simulink model "sensorExpoler_Encoder_Bourns"  (R2026a)
settings: Solver=FixedStepDiscrete  StopTime=32  FixedStep=0.0001
undefined symbols (not defined in the file): Blocking, Non
libraries: amg_usbconverter_n_connect_lib x2
settings Model: Creator=pboon  LastModifiedBy=matthurindo

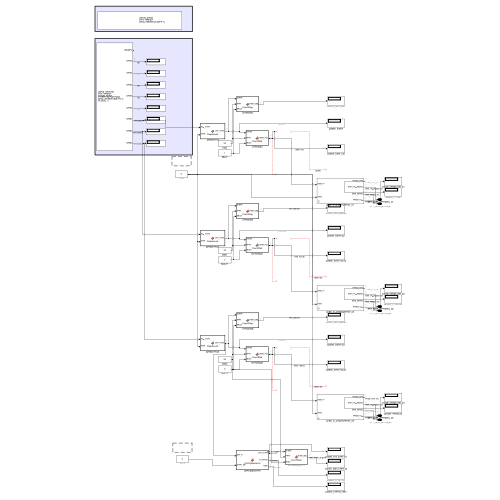
[thumbnail: Simulink's stored preview of the top-level diagram]
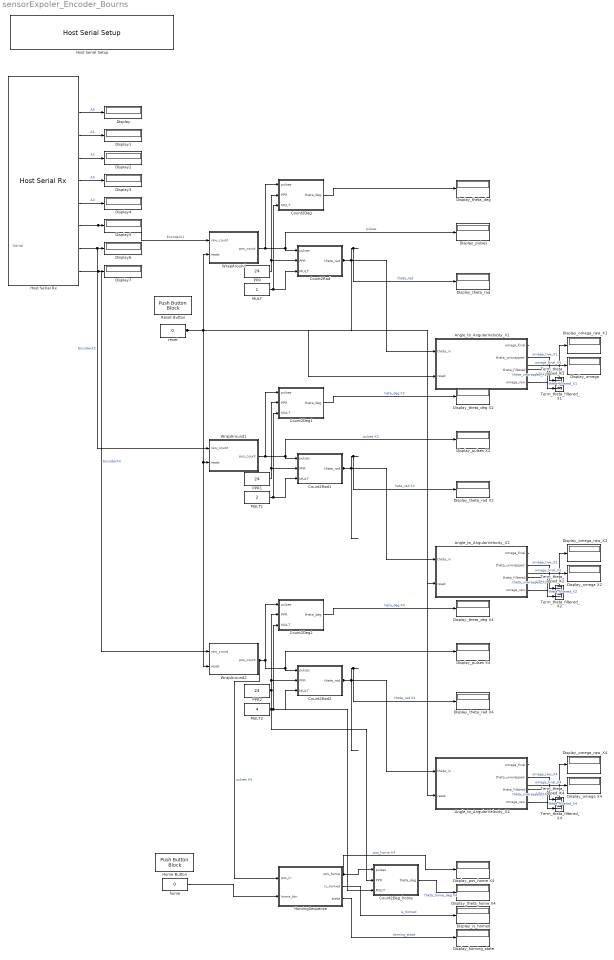
== system sensorExpoler_Encoder_Bourns ==
  note: Serial
  Angle_to_AngularVelocity_X1 : Subsystem  mask{Ts=0.001, fc_theta=0.5, fc_omega=5, Enable_velocity_filter=1, Enable_unwrap=0, Wrap_period=2*pi}
      mask prompts: Ts "Effective sensor sample time [s]"; fc_theta "Angle low-pass cutoff [Hz] (0 < fc < 1/(2*Ts))"; fc_omega "Velocity low-pass cutoff [Hz]"; Enable_velocity_filter "1 = light velocity LPF on, 0 = bypass"; Enable_unwrap "1 = unwrap a wrapped angle, 0 = angle already accumulated"; Wrap_period "Wrap period [rad] (2*pi) or [deg] (360)"
      mask help:
      | Filtered angle -> angular velocity (X1).
      | theta -> [unwrap] -> [1st-order angle LPF @ fc_theta] -> [(theta[k]-theta[k-1])/Ts] -> [light velocity LPF @ fc_omega] -> omega.
      | State initialised from the first valid sample; output 0 on first sample/reset.
  Angle_to_AngularVelocity_X2 : Subsystem  mask{Ts=0.001, fc_theta=1, fc_omega=5, Enable_velocity_filter=1, Enable_unwrap=0, Wrap_period=2*pi}
      mask prompts: Ts "Effective sensor sample time [s]"; fc_theta "Angle low-pass cutoff [Hz] (0 < fc < 1/(2*Ts))"; fc_omega "Velocity low-pass cutoff [Hz]"; Enable_velocity_filter "1 = light velocity LPF on, 0 = bypass"; Enable_unwrap "1 = unwrap a wrapped angle, 0 = angle already accumulated"; Wrap_period "Wrap period [rad] (2*pi) or [deg] (360)"
      mask help:
      | Filtered angle -> angular velocity (X2).
      | theta -> [unwrap] -> [1st-order angle LPF @ fc_theta] -> [(theta[k]-theta[k-1])/Ts] -> [light velocity LPF @ fc_omega] -> omega.
      | State initialised from the first valid sample; output 0 on first sample/reset.
  Angle_to_AngularVelocity_X4 : Subsystem  mask{Ts=0.001, fc_theta=2, fc_omega=5, Enable_velocity_filter=1, Enable_unwrap=0, Wrap_period=2*pi}
      mask prompts: Ts "Effective sensor sample time [s]"; fc_theta "Angle low-pass cutoff [Hz] (0 < fc < 1/(2*Ts))"; fc_omega "Velocity low-pass cutoff [Hz]"; Enable_velocity_filter "1 = light velocity LPF on, 0 = bypass"; Enable_unwrap "1 = unwrap a wrapped angle, 0 = angle already accumulated"; Wrap_period "Wrap period [rad] (2*pi) or [deg] (360)"
      mask help:
      | Filtered angle -> angular velocity (X4).
      | theta -> [unwrap] -> [1st-order angle LPF @ fc_theta] -> [(theta[k]-theta[k-1])/Ts] -> [light velocity LPF @ fc_omega] -> omega.
      | State initialised from the first valid sample; output 0 on first sample/reset.
  Count2Deg : MATLAB Function  TreatAsAtomicUnit=on
  Count2Deg1 : MATLAB Function  TreatAsAtomicUnit=on
  Count2Deg2 : MATLAB Function  TreatAsAtomicUnit=on
  Count2Deg_home : MATLAB Function  TreatAsAtomicUnit=on
  Count2Rad : MATLAB Function  TreatAsAtomicUnit=on
  Count2Rad1 : MATLAB Function  TreatAsAtomicUnit=on
  Count2Rad2 : MATLAB Function  TreatAsAtomicUnit=on
  Display{,1..7} (8 alike) : Display
  Display_homing_state : Display
  Display_is_homed : Display
  Display_omega : Display
  Display_omega X2 : Display
  Display_omega X4 : Display
  Display_omega_raw_X1 : Display
  Display_omega_raw_X2 : Display
  Display_omega_raw_X4 : Display
  Display_pos_home X4 : Display
  Display_pulses : Display
  Display_pulses X2 : Display
  Display_pulses X4 : Display
  Display_theta_deg : Display
  Display_theta_deg X2 : Display
  Display_theta_deg X4 : Display
  Display_theta_home X4 : Display
  Display_theta_rad : Display
  Display_theta_rad X2 : Display
  Display_theta_rad X4 : Display
  Home Button : PushButtonBlock  ButtonText=Home  IconOnColor=[0.0, 0.39215686274509803, 0.0]  IconOffColor=[0.0, 1.0, 0.0]  OffValue=0.000000
  HomingSequence : MATLAB Function  TreatAsAtomicUnit=on
  Host Serial Rx : amg_usbconverter_n_connect_lib/Host Serial Rx  conf=rx  port=<auto>  baudrate=2000000  databits=8  parity=None  stopbit=1  flowcontrol=None  transfer=Non-Blocking  timeout=5  packetmode=Binary  enableinitialvalues=off  initialvalues=[]  binheader='25'  binterminator='4E 4E'  porttype_double=0  porttype_single=0  porttype_int8=0  porttype_uint8=0  porttype_int16=0  porttype_uint16=5  porttype_int32=0  porttype_uint32=3  asciiformat='%d,%f'  rx_asciiterminator="CRLF (0x0D 0x0A - \"\\r\\n\")"  tx_asciiterminator="CRLF (0x0D 0x0A - \"\\r\\n\")"  sampletime=0.001  enablecustomportlabel=off  cinputportlabel=0  coutputportlabel=A  portpinstr=0  blockid=HostSerialRx  inputporttype=[]  inputportwidth=[]  inputportlabel={}  outputporttype=[3 5 5 5 5 5 7 7 7]  outputportwidth=[1 1 1 1 1 1 1 1 1]  outputportlabel={'READY','uint16','uint16','uint16','uint16','uint16','uint32','uint32','uint32'}  compat=0  optionstring=[]  autoport='<empty>'
  Host Serial Setup : amg_usbconverter_n_connect_lib/Host Serial Setup  conf=setup  port=<auto>  baudrate=2000000  databits=8  parity=None  stopbit=1  flowcontrol=None  transfer=Blocking  timeout=2  packetmode=Binary  initialvalues=[]  binheader='7E 7E'  binterminator='03 03'  porttype_double=0  porttype_single=1  porttype_int8=0  porttype_uint8=0  porttype_int16=0  porttype_uint16=0  porttype_int32=0  porttype_uint32=2  asciiformat='%d %u %x'  rx_asciiterminator="CRLF (0x0D 0x0A - \"\\r\\n\")"  tx_asciiterminator="CRLF (0x0D 0x0A - \"\\r\\n\")"  sampletime=-1  enablecustomportlabel=off  cinputportlabel=0  coutputportlabel=A  portpinstr=0  blockid=HostSerialSetup  inputporttype=[]  inputportwidth=[]  inputportlabel={}  outputporttype=[]  outputportwidth=[]  outputportlabel={}  compat=0  optionstring=[]  autoport='<empty>'
  MULT : Constant
  MULT1 : Constant  Value=2
  MULT2 : Constant  Value=4
  PPR : Constant  Value=24
  PPR1 : Constant  Value=24
  PPR2 : Constant  Value=24
  Reset Button : PushButtonBlock  IconOnColor=[0.0, 0.39215686274509803, 0.0]  IconOffColor=[0.0, 1.0, 0.0]  OffValue=0.000000
  Term_theta_filtered_X1 : Terminator
  Term_theta_filtered_X2 : Terminator
  Term_theta_filtered_X4 : Terminator
  Term_theta_unwrapped_X1 : Terminator
  Term_theta_unwrapped_X2 : Terminator
  Term_theta_unwrapped_X4 : Terminator
  WrapAround : MATLAB Function  TreatAsAtomicUnit=on
  WrapAround1 : MATLAB Function  TreatAsAtomicUnit=on
  WrapAround2 : MATLAB Function  TreatAsAtomicUnit=on
  home : Constant  Value=0
  reset : Constant  Value=0
  wires:
  Host Serial Rx/2 -> Display/1  "A0"
  Host Serial Rx/3 -> Display1/1  "A1"
  Host Serial Rx/4 -> Display2/1  "A2"
  Host Serial Rx/5 -> Display3/1  "A3"
  Host Serial Rx/6 -> Display4/1  "A4"
  Host Serial Rx/7 -> WrapAround/1(raw_count), Display5/1  "EncoderX1"
  Host Serial Rx/8 -> WrapAround1/1(raw_count), Display6/1  "EncoderX2"
  Host Serial Rx/9 -> WrapAround2/1(raw_count), Display7/1  "EncoderX4"
  reset/1 -> WrapAround/2(reset), WrapAround1/2(reset), WrapAround2/2(reset), Angle_to_AngularVelocity_X1/2(reset), Angle_to_AngularVelocity_X2/2(reset), Angle_to_AngularVelocity_X4/2(reset)
  PPR/1 -> Count2Rad/2(PPR), Count2Deg/2(PPR)
  MULT/1 -> Count2Rad/3(MULT), Count2Deg/3(MULT)
  WrapAround/1(pos_count) -> Count2Rad/1(pulses), Display_pulses/1, Count2Deg/1(pulses)  "pulses"
  Count2Rad/1(theta_rad) -> Display_theta_rad/1, Angle_to_AngularVelocity_X1/1(theta_in)  "theta_rad"
  Count2Deg/1(theta_deg) -> Display_theta_deg/1
  ? -> ?  "dtheta"
  ? -> ?  "dtheta X2"
  WrapAround1/1(pos_count) -> Count2Rad1/1(pulses), Display_pulses X2/1, Count2Deg1/1(pulses)  "pulses X2"
  MULT1/1 -> Count2Rad1/3(MULT), Count2Deg1/3(MULT)
  Count2Rad1/1(theta_rad) -> Display_theta_rad X2/1, Angle_to_AngularVelocity_X2/1(theta_in)  "heta_rad X2"
  Count2Deg1/1(theta_deg) -> Display_theta_deg X2/1  "heta_deg X2"
  PPR1/1 -> Count2Rad1/2(PPR), Count2Deg1/2(PPR)
  ? -> ?  "dtheta X4"
  WrapAround2/1(pos_count) -> Count2Rad2/1(pulses), Display_pulses X4/1, Count2Deg2/1(pulses), HomingSequence/1(pos_in)  "pulses X4"
  MULT2/1 -> Count2Rad2/3(MULT), Count2Deg2/3(MULT), Count2Deg_home/3(MULT)
  Count2Rad2/1(theta_rad) -> Display_theta_rad X4/1, Angle_to_AngularVelocity_X4/1(theta_in)  "theta_rad X4"
  Count2Deg2/1(theta_deg) -> Display_theta_deg X4/1  "heta_deg X4"
  PPR2/1 -> Count2Rad2/2(PPR), Count2Deg2/2(PPR), Count2Deg_home/2(PPR)
  Angle_to_AngularVelocity_X1/1(omega_final) -> Display_omega/1  "omega_final_X1"
  Angle_to_AngularVelocity_X1/4(omega_raw) -> Display_omega_raw_X1/1  "omega_raw_X1"
  Angle_to_AngularVelocity_X1/2(theta_unwrapped) -> Term_theta_unwrapped_X1/1  "theta_unwrapped_X1"
  Angle_to_AngularVelocity_X1/3(theta_filtered) -> Term_theta_filtered_X1/1  "theta_filtered_X1"
  Angle_to_AngularVelocity_X2/1(omega_final) -> Display_omega X2/1  "omega_final_X2"
  Angle_to_AngularVelocity_X2/4(omega_raw) -> Display_omega_raw_X2/1  "omega_raw_X2"
  Angle_to_AngularVelocity_X2/2(theta_unwrapped) -> Term_theta_unwrapped_X2/1  "theta_unwrapped_X2"
  Angle_to_AngularVelocity_X2/3(theta_filtered) -> Term_theta_filtered_X2/1  "theta_filtered_X2"
  Angle_to_AngularVelocity_X4/1(omega_final) -> Display_omega X4/1  "omega_final_X4"
  Angle_to_AngularVelocity_X4/4(omega_raw) -> Display_omega_raw_X4/1  "omega_raw_X4"
  Angle_to_AngularVelocity_X4/2(theta_unwrapped) -> Term_theta_unwrapped_X4/1  "theta_unwrapped_X4"
  Angle_to_AngularVelocity_X4/3(theta_filtered) -> Term_theta_filtered_X4/1  "theta_filtered_X4"
  home/1 -> HomingSequence/2(home_btn)
  HomingSequence/1(pos_home) -> Count2Deg_home/1(pulses), Display_pos_home X4/1  "pos_home X4"
  Count2Deg_home/1(theta_deg) -> Display_theta_home X4/1  "theta_home_deg X4"
  HomingSequence/2(is_homed) -> Display_is_homed/1  "is_homed"
  HomingSequence/3(state) -> Display_homing_state/1  "homing_state"

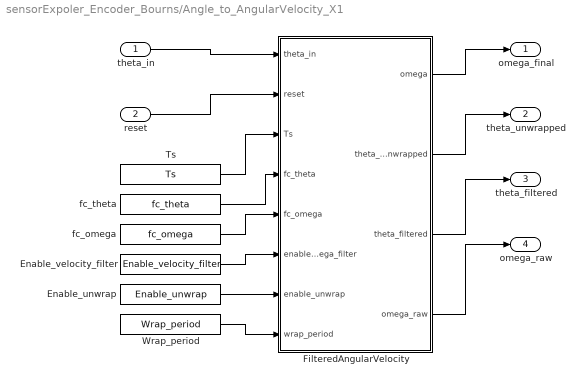
== system sensorExpoler_Encoder_Bourns/Angle_to_AngularVelocity_X1 ==
  theta_in : Inport
  reset : Inport  Port=2
  Enable_unwrap : Constant  Value=Enable_unwrap
  Enable_velocity_filter : Constant  Value=Enable_velocity_filter
  FilteredAngularVelocity : MATLAB Function  TreatAsAtomicUnit=on
  Ts : Constant  Value=Ts
  Wrap_period : Constant  Value=Wrap_period
  fc_omega : Constant  Value=fc_omega
  fc_theta : Constant  Value=fc_theta
  omega_final : Outport
  theta_unwrapped : Outport  Port=2
  theta_filtered : Outport  Port=3
  omega_raw : Outport  Port=4
  wires:
  theta_in/1 -> FilteredAngularVelocity/1(theta_in)
  reset/1 -> FilteredAngularVelocity/2(reset)
  Ts/1 -> FilteredAngularVelocity/3(Ts)
  fc_theta/1 -> FilteredAngularVelocity/4(fc_theta)
  fc_omega/1 -> FilteredAngularVelocity/5(fc_omega)
  Enable_velocity_filter/1 -> FilteredAngularVelocity/6(enable_omega_filter)
  Enable_unwrap/1 -> FilteredAngularVelocity/7(enable_unwrap)
  Wrap_period/1 -> FilteredAngularVelocity/8(wrap_period)
  FilteredAngularVelocity/1(omega) -> omega_final/1
  FilteredAngularVelocity/2(theta_unwrapped) -> theta_unwrapped/1
  FilteredAngularVelocity/3(theta_filtered) -> theta_filtered/1
  FilteredAngularVelocity/4(omega_raw) -> omega_raw/1

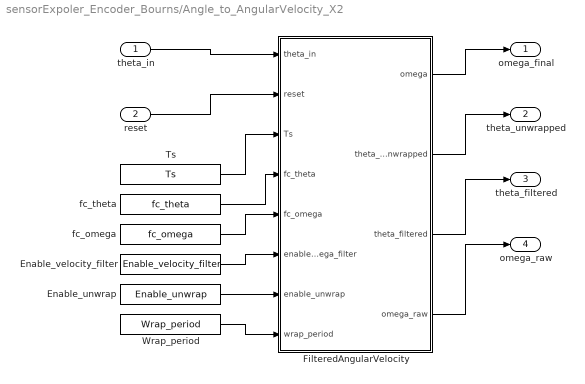
== system sensorExpoler_Encoder_Bourns/Angle_to_AngularVelocity_X2 ==
  theta_in : Inport
  reset : Inport  Port=2
  Enable_unwrap : Constant  Value=Enable_unwrap
  Enable_velocity_filter : Constant  Value=Enable_velocity_filter
  FilteredAngularVelocity : MATLAB Function  TreatAsAtomicUnit=on
  Ts : Constant  Value=Ts
  Wrap_period : Constant  Value=Wrap_period
  fc_omega : Constant  Value=fc_omega
  fc_theta : Constant  Value=fc_theta
  omega_final : Outport
  theta_unwrapped : Outport  Port=2
  theta_filtered : Outport  Port=3
  omega_raw : Outport  Port=4
  wires:
  theta_in/1 -> FilteredAngularVelocity/1(theta_in)
  reset/1 -> FilteredAngularVelocity/2(reset)
  Ts/1 -> FilteredAngularVelocity/3(Ts)
  fc_theta/1 -> FilteredAngularVelocity/4(fc_theta)
  fc_omega/1 -> FilteredAngularVelocity/5(fc_omega)
  Enable_velocity_filter/1 -> FilteredAngularVelocity/6(enable_omega_filter)
  Enable_unwrap/1 -> FilteredAngularVelocity/7(enable_unwrap)
  Wrap_period/1 -> FilteredAngularVelocity/8(wrap_period)
  FilteredAngularVelocity/1(omega) -> omega_final/1
  FilteredAngularVelocity/2(theta_unwrapped) -> theta_unwrapped/1
  FilteredAngularVelocity/3(theta_filtered) -> theta_filtered/1
  FilteredAngularVelocity/4(omega_raw) -> omega_raw/1

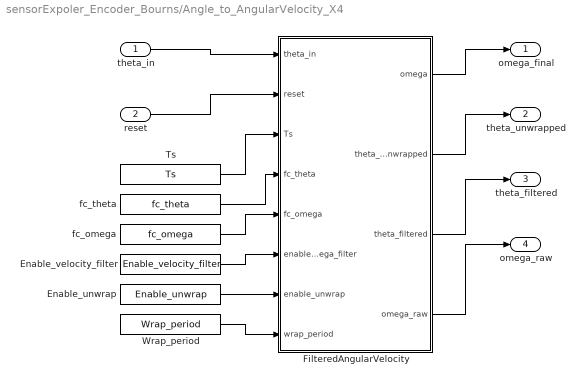
== system sensorExpoler_Encoder_Bourns/Angle_to_AngularVelocity_X4 ==
  theta_in : Inport
  reset : Inport  Port=2
  Enable_unwrap : Constant  Value=Enable_unwrap
  Enable_velocity_filter : Constant  Value=Enable_velocity_filter
  FilteredAngularVelocity : MATLAB Function  TreatAsAtomicUnit=on
  Ts : Constant  Value=Ts
  Wrap_period : Constant  Value=Wrap_period
  fc_omega : Constant  Value=fc_omega
  fc_theta : Constant  Value=fc_theta
  omega_final : Outport
  theta_unwrapped : Outport  Port=2
  theta_filtered : Outport  Port=3
  omega_raw : Outport  Port=4
  wires:
  theta_in/1 -> FilteredAngularVelocity/1(theta_in)
  reset/1 -> FilteredAngularVelocity/2(reset)
  Ts/1 -> FilteredAngularVelocity/3(Ts)
  fc_theta/1 -> FilteredAngularVelocity/4(fc_theta)
  fc_omega/1 -> FilteredAngularVelocity/5(fc_omega)
  Enable_velocity_filter/1 -> FilteredAngularVelocity/6(enable_omega_filter)
  Enable_unwrap/1 -> FilteredAngularVelocity/7(enable_unwrap)
  Wrap_period/1 -> FilteredAngularVelocity/8(wrap_period)
  FilteredAngularVelocity/1(omega) -> omega_final/1
  FilteredAngularVelocity/2(theta_unwrapped) -> theta_unwrapped/1
  FilteredAngularVelocity/3(theta_filtered) -> theta_filtered/1
  FilteredAngularVelocity/4(omega_raw) -> omega_raw/1

== matlab function sensorExpoler_Encoder_Bourns/Count2Deg2 ==
  data: pulses input; theta_deg output; PPR input; MULT input
function theta_deg = Count2Deg(pulses, PPR, MULT)
theta_deg = (pulses / (PPR * MULT)) * 360;

== matlab function sensorExpoler_Encoder_Bourns/Count2Rad2 ==
  data: pulses input; theta_rad output; PPR input; MULT input
function theta_rad = Count2Rad(pulses, PPR, MULT)
theta_rad = (pulses / (PPR * MULT)) * 2*pi;

== matlab function sensorExpoler_Encoder_Bourns/Angle_to_AngularVelocity_X4/FilteredAngularVelocity ==
  data: theta_in input; omega output; reset input; Ts input; fc_theta input; fc_omega input; enable_omega_filter input; enable_unwrap input; wrap_period input; theta_unwrapped output; theta_filtered output; omega_raw output
function [omega, theta_unwrapped, theta_filtered, omega_raw] = FilteredAngularVelocity(theta_in, reset, Ts, fc_theta, fc_omega, enable_omega_filter, enable_unwrap, wrap_period)
%#codegen
% FilteredAngularVelocity -- causal angle-to-angular-velocity pipeline.
%
%   [omega, theta_unwrapped, theta_filtered, omega_raw] = ...
%       FilteredAngularVelocity(theta_in, reset, Ts, fc_theta, fc_omega, ...
%                               enable_omega_filter, enable_unwrap, wrap_period)
%
% Pipeline (matches the task specification):
%   theta_in -> [unwrap, if enabled] -> [1st-order LPF @ fc_theta]
%            -> [backward difference / Ts] -> [optional LPF @ fc_omega] -> omega
%
% Inputs
%   theta_in           : angle [rad].  If it comes from WrapAround/Count2Rad
%                        it is ALREADY an accumulated (unwrapped) position,
%                        so leave enable_unwrap = false.  Set true only when
%                        theta_in itself wraps.
%   reset              : ~= 0 re-initialises every state from theta_in and
%                        outputs omega = 0 (no spike after a counter reset).
%   Ts                 : effective sensor update interval [s] (1 ms here).
%   fc_theta           : angle LPF cutoff [Hz], 0 < fc_theta < 1/(2*Ts).
%   fc_omega           : velocity LPF cutoff [Hz] (used only if enabled).
%   enable_omega_filter: true/false, bypass for the light velocity LPF.
%   enable_unwrap      : true/false, stateful unwrap of a wrapped angle.
%   wrap_period        : wrap period [rad] (2*pi) or [deg] (360).
%
% Outputs
%   omega              : final angular velocity [rad/s].
%   theta_unwrapped    : angle after the (optional) unwrap [rad].
%   theta_filtered     : angle after the causal LPF [rad] (diagnostic).
%   omega_raw          : velocity BEFORE the optional velocity LPF [rad/s].
%
% Initialisation / startup behaviour
%   On the first valid sample (or right after reset) every state is set to
%   theta_in and omega is forced to 0, so no artificial startup impulse and
%   no drift from an implicit zero initial condition.
%
% Causality / timing
%   Pure sample-by-sample processing at Ts.  No gradient()/zero-phase
%   filtering; safe for live Simulink execution and code generation.

persistent prev_raw prev_unwrapped theta_f prev_theta_f omega_f initialised

if isempty(initialised)
    initialised = false;
    prev_raw = 0; prev_unwrapped = 0; theta_f = 0; prev_theta_f = 0; omega_f = 0;
end

valid = isfinite(theta_in);

if ~valid
    % Hold the last outputs; do not let a bad sample corrupt the state.
    omega = omega_f; theta_unwrapped = prev_unwrapped;
    theta_filtered = theta_f; omega_raw = 0;
    return
end

if ~initialised || reset ~= 0
    % First valid sample or explicit re-zero: initialise from the sample.
    prev_raw       = theta_in;
    prev_unwrapped = theta_in;
    theta_f        = theta_in;
    prev_theta_f   = theta_in;
    omega_f        = 0;
    initialised    = true;
    omega = 0; theta_unwrapped = theta_in;
    theta_filtered = theta_in; omega_raw = 0;
    return
end

% ---- 1. unwrap only if the source itself wraps --------------------------
if enable_unwrap
    d = theta_in - prev_raw;
    if d > wrap_period/2
        d = d - wrap_period;
    elseif d < -wrap_period/2
        d = d + wrap_period;
    end
    theta_unwrapped = prev_unwrapped + d;
else
    theta_unwrapped = theta_in;   % already an accumulated position
end

% ---- 2. causal first-order low-pass filter on the angle ------------------
alpha_theta = exp(-2*pi*fc_theta*Ts);
theta_f = alpha_theta*theta_f + (1 - alpha_theta)*theta_unwrapped;

% ---- 3. discrete backward difference of the filtered angle ---------------
omega_raw = (theta_f - prev_theta_f) / Ts;

% ---- 4. optional light low-pass filter on the velocity -------------------
if enable_omega_filter
    alpha_omega = exp(-2*pi*fc_omega*Ts);
    omega_f = alpha_omega*omega_f + (1 - alpha_omega)*omega_raw;
else
    omega_f = omega_raw;
end

% ---- state update ---------------------------------------------------------
prev_raw       = theta_in;
prev_unwrapped = theta_unwrapped;
prev_theta_f   = theta_f;
omega          = omega_f;
theta_filtered = theta_f;
end

== matlab function sensorExpoler_Encoder_Bourns/WrapAround2 ==
  data: raw_count input; pos_count output; reset input
function pos_count = WrapAround(raw_count, reset)
%#codegen
persistent prev acc nBlank
MAXC          = 65536;      % hardware counter modulus
HALF          = MAXC/2;
BLANK_SAMPLES = 150;

if isempty(prev) || isempty(acc) || isempty(nBlank)
    prev = 0; acc = 0; nBlank = 0;
end

rawd  = double(raw_count);
valid = isfinite(rawd);
raw   = mod(rawd, MAXC);          % NaN/Inf -> NaN, never used unless valid

% --- reset first, so it can't be swallowed by a bad sample ---
if reset ~= 0
    acc = 0;
    if valid
        prev   = raw;                 % re-latch immediately
        nBlank = BLANK_SAMPLES;       % skip re-blanking
    else
        nBlank = BLANK_SAMPLES - 1;   % next valid sample re-latches prev, no delta
    end
    pos_count = 0;  return
end

% --- reject invalid samples before they touch the state ---
if ~valid
    pos_count = acc;  return
end

% --- power-up blanking (also serves as the re-latch after an invalid reset) ---
if nBlank < BLANK_SAMPLES
    nBlank    = nBlank + 1;
    prev      = raw;
    pos_count = acc;  return
end

% --- unwrap ---
delta = raw - prev;
if delta >= HALF
    delta = delta - MAXC;
elseif delta < -HALF
    delta = delta + MAXC;
end
acc       = acc + delta;
prev      = raw;
pos_count = acc;
end

== matlab function sensorExpoler_Encoder_Bourns/HomingSequence ==
  data: pos_in input; pos_home output; home_btn input; is_homed output; state output
function [pos_home, is_homed, state] = HomingSequence(pos_in, home_btn)
%#codegen
% Homing for an incremental encoder with only A/B wired (no index pulse):
% turn the shaft to the home mark, press Home; the count becomes zero once
% the shaft has stayed still for STILL_N samples. state: 0 = not homed,
% 1 = waiting for standstill, 2 = homed. pos_in, pos_home in counts.
persistent st offset prevBtn anchor nStill
STILL_N   = 200;   % 200 ms at Ts = 1 ms
STILL_TOL = 1;     % counts
if isempty(st)
    st = 0; offset = 0; prevBtn = false; anchor = pos_in; nStill = 0;
end

btn = home_btn ~= 0;
if btn && ~prevBtn              % rising edge of Home: start (re)homing
    st = 1;  anchor = pos_in;  nStill = 0;
end
prevBtn = btn;

if abs(pos_in - anchor) <= STILL_TOL
    nStill = nStill + 1;        % shaft still
else
    anchor = pos_in;  nStill = 0;
end

if st == 1 && nStill >= STILL_N
    offset = pos_in;            % latch the home position
    st = 2;
end

pos_home = pos_in - offset;
is_homed = st == 2;
state    = st;
end

== matlab function sensorExpoler_Encoder_Bourns/Count2Deg_home ==
  data: pulses input; theta_deg output; PPR input; MULT input
function theta_deg = Count2Deg(pulses, PPR, MULT)
theta_deg = (pulses / (PPR * MULT)) * 360;

== matlab function sensorExpoler_Encoder_Bourns/Count2Rad ==
  data: pulses input; theta_rad output; PPR input; MULT input
function theta_rad = Count2Rad(pulses, PPR, MULT)
theta_rad = (pulses / (PPR * MULT)) * 2*pi;

== matlab function sensorExpoler_Encoder_Bourns/Count2Deg ==
  data: pulses input; theta_deg output; PPR input; MULT input
function theta_deg = Count2Deg(pulses, PPR, MULT)
theta_deg = (pulses / (PPR * MULT)) * 360;

== matlab function sensorExpoler_Encoder_Bourns/WrapAround ==
  data: raw_count input; pos_count output; reset input
function pos_count = WrapAround(raw_count, reset)
%#codegen
persistent prev acc nBlank
MAXC          = 65536;      % hardware counter modulus
HALF          = MAXC/2;
BLANK_SAMPLES = 150;

if isempty(prev) || isempty(acc) || isempty(nBlank)
    prev = 0; acc = 0; nBlank = 0;
end

rawd  = double(raw_count);
valid = isfinite(rawd);
raw   = mod(rawd, MAXC);          % NaN/Inf -> NaN, never used unless valid

% --- reset first, so it can't be swallowed by a bad sample ---
if reset ~= 0
    acc = 0;
    if valid
        prev   = raw;                 % re-latch immediately
        nBlank = BLANK_SAMPLES;       % skip re-blanking
    else
        nBlank = BLANK_SAMPLES - 1;   % next valid sample re-latches prev, no delta
    end
    pos_count = 0;  return
end

% --- reject invalid samples before they touch the state ---
if ~valid
    pos_count = acc;  return
end

% --- power-up blanking (also serves as the re-latch after an invalid reset) ---
if nBlank < BLANK_SAMPLES
    nBlank    = nBlank + 1;
    prev      = raw;
    pos_count = acc;  return
end

% --- unwrap ---
delta = raw - prev;
if delta >= HALF
    delta = delta - MAXC;
elseif delta < -HALF
    delta = delta + MAXC;
end
acc       = acc + delta;
prev      = raw;
pos_count = acc;
end

== matlab function sensorExpoler_Encoder_Bourns/Angle_to_AngularVelocity_X1/FilteredAngularVelocity ==
  data: theta_in input; omega output; reset input; Ts input; fc_theta input; fc_omega input; enable_omega_filter input; enable_unwrap input; wrap_period input; theta_unwrapped output; theta_filtered output; omega_raw output
function [omega, theta_unwrapped, theta_filtered, omega_raw] = FilteredAngularVelocity(theta_in, reset, Ts, fc_theta, fc_omega, enable_omega_filter, enable_unwrap, wrap_period)
%#codegen
% FilteredAngularVelocity -- causal angle-to-angular-velocity pipeline.
%
%   [omega, theta_unwrapped, theta_filtered, omega_raw] = ...
%       FilteredAngularVelocity(theta_in, reset, Ts, fc_theta, fc_omega, ...
%                               enable_omega_filter, enable_unwrap, wrap_period)
%
% Pipeline (matches the task specification):
%   theta_in -> [unwrap, if enabled] -> [1st-order LPF @ fc_theta]
%            -> [backward difference / Ts] -> [optional LPF @ fc_omega] -> omega
%
% Inputs
%   theta_in           : angle [rad].  If it comes from WrapAround/Count2Rad
%                        it is ALREADY an accumulated (unwrapped) position,
%                        so leave enable_unwrap = false.  Set true only when
%                        theta_in itself wraps.
%   reset              : ~= 0 re-initialises every state from theta_in and
%                        outputs omega = 0 (no spike after a counter reset).
%   Ts                 : effective sensor update interval [s] (1 ms here).
%   fc_theta           : angle LPF cutoff [Hz], 0 < fc_theta < 1/(2*Ts).
%   fc_omega           : velocity LPF cutoff [Hz] (used only if enabled).
%   enable_omega_filter: true/false, bypass for the light velocity LPF.
%   enable_unwrap      : true/false, stateful unwrap of a wrapped angle.
%   wrap_period        : wrap period [rad] (2*pi) or [deg] (360).
%
% Outputs
%   omega              : final angular velocity [rad/s].
%   theta_unwrapped    : angle after the (optional) unwrap [rad].
%   theta_filtered     : angle after the causal LPF [rad] (diagnostic).
%   omega_raw          : velocity BEFORE the optional velocity LPF [rad/s].
%
% Initialisation / startup behaviour
%   On the first valid sample (or right after reset) every state is set to
%   theta_in and omega is forced to 0, so no artificial startup impulse and
%   no drift from an implicit zero initial condition.
%
% Causality / timing
%   Pure sample-by-sample processing at Ts.  No gradient()/zero-phase
%   filtering; safe for live Simulink execution and code generation.

persistent prev_raw prev_unwrapped theta_f prev_theta_f omega_f initialised

if isempty(initialised)
    initialised = false;
    prev_raw = 0; prev_unwrapped = 0; theta_f = 0; prev_theta_f = 0; omega_f = 0;
end

valid = isfinite(theta_in);

if ~valid
    % Hold the last outputs; do not let a bad sample corrupt the state.
    omega = omega_f; theta_unwrapped = prev_unwrapped;
    theta_filtered = theta_f; omega_raw = 0;
    return
end

if ~initialised || reset ~= 0
    % First valid sample or explicit re-zero: initialise from the sample.
    prev_raw       = theta_in;
    prev_unwrapped = theta_in;
    theta_f        = theta_in;
    prev_theta_f   = theta_in;
    omega_f        = 0;
    initialised    = true;
    omega = 0; theta_unwrapped = theta_in;
    theta_filtered = theta_in; omega_raw = 0;
    return
end

% ---- 1. unwrap only if the source itself wraps --------------------------
if enable_unwrap
    d = theta_in - prev_raw;
    if d > wrap_period/2
        d = d - wrap_period;
    elseif d < -wrap_period/2
        d = d + wrap_period;
    end
    theta_unwrapped = prev_unwrapped + d;
else
    theta_unwrapped = theta_in;   % already an accumulated position
end

% ---- 2. causal first-order low-pass filter on the angle ------------------
alpha_theta = exp(-2*pi*fc_theta*Ts);
theta_f = alpha_theta*theta_f + (1 - alpha_theta)*theta_unwrapped;

% ---- 3. discrete backward difference of the filtered angle ---------------
omega_raw = (theta_f - prev_theta_f) / Ts;

% ---- 4. optional light low-pass filter on the velocity -------------------
if enable_omega_filter
    alpha_omega = exp(-2*pi*fc_omega*Ts);
    omega_f = alpha_omega*omega_f + (1 - alpha_omega)*omega_raw;
else
    omega_f = omega_raw;
end

% ---- state update ---------------------------------------------------------
prev_raw       = theta_in;
prev_unwrapped = theta_unwrapped;
prev_theta_f   = theta_f;
omega          = omega_f;
theta_filtered = theta_f;
end

== matlab function sensorExpoler_Encoder_Bourns/Count2Deg1 ==
  data: pulses input; theta_deg output; PPR input; MULT input
function theta_deg = Count2Deg(pulses, PPR, MULT)
theta_deg = (pulses / (PPR * MULT)) * 360;

== matlab function sensorExpoler_Encoder_Bourns/Count2Rad1 ==
  data: pulses input; theta_rad output; PPR input; MULT input
function theta_rad = Count2Rad(pulses, PPR, MULT)
theta_rad = (pulses / (PPR * MULT)) * 2*pi;

== matlab function sensorExpoler_Encoder_Bourns/Angle_to_AngularVelocity_X2/FilteredAngularVelocity ==
  data: theta_in input; omega output; reset input; Ts input; fc_theta input; fc_omega input; enable_omega_filter input; enable_unwrap input; wrap_period input; theta_unwrapped output; theta_filtered output; omega_raw output
function [omega, theta_unwrapped, theta_filtered, omega_raw] = FilteredAngularVelocity(theta_in, reset, Ts, fc_theta, fc_omega, enable_omega_filter, enable_unwrap, wrap_period)
%#codegen
% FilteredAngularVelocity -- causal angle-to-angular-velocity pipeline.
%
%   [omega, theta_unwrapped, theta_filtered, omega_raw] = ...
%       FilteredAngularVelocity(theta_in, reset, Ts, fc_theta, fc_omega, ...
%                               enable_omega_filter, enable_unwrap, wrap_period)
%
% Pipeline (matches the task specification):
%   theta_in -> [unwrap, if enabled] -> [1st-order LPF @ fc_theta]
%            -> [backward difference / Ts] -> [optional LPF @ fc_omega] -> omega
%
% Inputs
%   theta_in           : angle [rad].  If it comes from WrapAround/Count2Rad
%                        it is ALREADY an accumulated (unwrapped) position,
%                        so leave enable_unwrap = false.  Set true only when
%                        theta_in itself wraps.
%   reset              : ~= 0 re-initialises every state from theta_in and
%                        outputs omega = 0 (no spike after a counter reset).
%   Ts                 : effective sensor update interval [s] (1 ms here).
%   fc_theta           : angle LPF cutoff [Hz], 0 < fc_theta < 1/(2*Ts).
%   fc_omega           : velocity LPF cutoff [Hz] (used only if enabled).
%   enable_omega_filter: true/false, bypass for the light velocity LPF.
%   enable_unwrap      : true/false, stateful unwrap of a wrapped angle.
%   wrap_period        : wrap period [rad] (2*pi) or [deg] (360).
%
% Outputs
%   omega              : final angular velocity [rad/s].
%   theta_unwrapped    : angle after the (optional) unwrap [rad].
%   theta_filtered     : angle after the causal LPF [rad] (diagnostic).
%   omega_raw          : velocity BEFORE the optional velocity LPF [rad/s].
%
% Initialisation / startup behaviour
%   On the first valid sample (or right after reset) every state is set to
%   theta_in and omega is forced to 0, so no artificial startup impulse and
%   no drift from an implicit zero initial condition.
%
% Causality / timing
%   Pure sample-by-sample processing at Ts.  No gradient()/zero-phase
%   filtering; safe for live Simulink execution and code generation.

persistent prev_raw prev_unwrapped theta_f prev_theta_f omega_f initialised

if isempty(initialised)
    initialised = false;
    prev_raw = 0; prev_unwrapped = 0; theta_f = 0; prev_theta_f = 0; omega_f = 0;
end

valid = isfinite(theta_in);

if ~valid
    % Hold the last outputs; do not let a bad sample corrupt the state.
    omega = omega_f; theta_unwrapped = prev_unwrapped;
    theta_filtered = theta_f; omega_raw = 0;
    return
end

if ~initialised || reset ~= 0
    % First valid sample or explicit re-zero: initialise from the sample.
    prev_raw       = theta_in;
    prev_unwrapped = theta_in;
    theta_f        = theta_in;
    prev_theta_f   = theta_in;
    omega_f        = 0;
    initialised    = true;
    omega = 0; theta_unwrapped = theta_in;
    theta_filtered = theta_in; omega_raw = 0;
    return
end

% ---- 1. unwrap only if the source itself wraps --------------------------
if enable_unwrap
    d = theta_in - prev_raw;
    if d > wrap_period/2
        d = d - wrap_period;
    elseif d < -wrap_period/2
        d = d + wrap_period;
    end
    theta_unwrapped = prev_unwrapped + d;
else
    theta_unwrapped = theta_in;   % already an accumulated position
end

% ---- 2. causal first-order low-pass filter on the angle ------------------
alpha_theta = exp(-2*pi*fc_theta*Ts);
theta_f = alpha_theta*theta_f + (1 - alpha_theta)*theta_unwrapped;

% ---- 3. discrete backward difference of the filtered angle ---------------
omega_raw = (theta_f - prev_theta_f) / Ts;

% ---- 4. optional light low-pass filter on the velocity -------------------
if enable_omega_filter
    alpha_omega = exp(-2*pi*fc_omega*Ts);
    omega_f = alpha_omega*omega_f + (1 - alpha_omega)*omega_raw;
else
    omega_f = omega_raw;
end

% ---- state update ---------------------------------------------------------
prev_raw       = theta_in;
prev_unwrapped = theta_unwrapped;
prev_theta_f   = theta_f;
omega          = omega_f;
theta_filtered = theta_f;
end

== matlab function sensorExpoler_Encoder_Bourns/WrapAround1 ==
  data: raw_count input; pos_count output; reset input
function pos_count = WrapAround(raw_count, reset)
%#codegen
persistent prev acc nBlank
MAXC          = 65536;      % hardware counter modulus
HALF          = MAXC/2;
BLANK_SAMPLES = 150;

if isempty(prev) || isempty(acc) || isempty(nBlank)
    prev = 0; acc = 0; nBlank = 0;
end

rawd  = double(raw_count);
valid = isfinite(rawd);
raw   = mod(rawd, MAXC);          % NaN/Inf -> NaN, never used unless valid

% --- reset first, so it can't be swallowed by a bad sample ---
if reset ~= 0
    acc = 0;
    if valid
        prev   = raw;                 % re-latch immediately
        nBlank = BLANK_SAMPLES;       % skip re-blanking
    else
        nBlank = BLANK_SAMPLES - 1;   % next valid sample re-latches prev, no delta
    end
    pos_count = 0;  return
end

% --- reject invalid samples before they touch the state ---
if ~valid
    pos_count = acc;  return
end

% --- power-up blanking (also serves as the re-latch after an invalid reset) ---
if nBlank < BLANK_SAMPLES
    nBlank    = nBlank + 1;
    prev      = raw;
    pos_count = acc;  return
end

% --- unwrap ---
delta = raw - prev;
if delta >= HALF
    delta = delta - MAXC;
elseif delta < -HALF
    delta = delta + MAXC;
end
acc       = acc + delta;
prev      = raw;
pos_count = acc;
end
